simulink model "PruebaSDRRX"  (R2025b)
settings: Solver=VariableStepAuto  StartTime=0.0  StopTime=30  RelTol=1e-3
undefined symbols (not defined in the file or in its folder): gray, RX, TX
libraries: commdigbbndpm3 x1, commfilt2 x1, commsdrhw_v2 x1
settings Model: Creator=JuanDiego  LastModifiedBy=juand

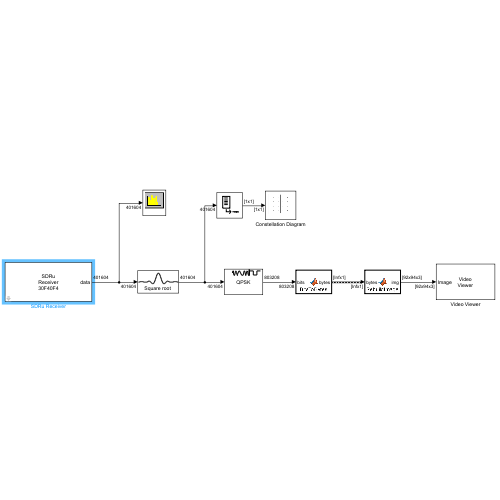
[thumbnail: Simulink's stored preview of the top-level diagram]
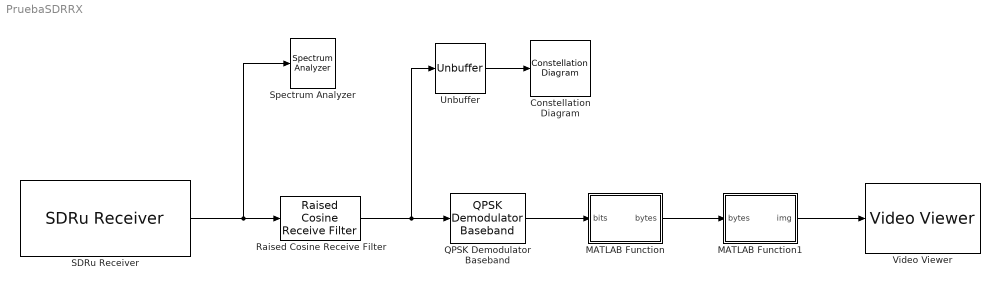
== system PruebaSDRRX ==
  Constellation Diagram : ConstellationDiagram  WindowPosition=[695.000000,130.000000,600.000000,582.000000,]  ScopeFrameLocation=window  SymbolsToDisplaySource=Property  SymbolsToDisplay=5000  ReferenceConstellation=QPSK
  MATLAB Function : MATLAB Function  TreatAsAtomicUnit=on
  MATLAB Function1 : MATLAB Function  TreatAsAtomicUnit=on
  QPSK Demodulator Baseband : commdigbbndpm3/QPSK Demodulator Baseband  OutType=Bit  DecType=Hard decision  VarSource=Dialog  Variance=1  Dec=Gray  Ph=pi/4  outDtype1=double  outDtype2=Inherit via internal rule  derotateFactorWordLen=16  derotateFactorDataTypeStr=Inherit: Same word length as input  derotateFactorLastDataTypeStr=Inherit: Same word length as input
  Raised Cosine Receive Filter : commfilt2/Raised Cosine Receive Filter  filtType=Square root  R=0.25  filtSpan=8  N=8  downFactor=1  downOffset=0  filterGain=1  InputProcessing=Columns as channels (frame based)  RateOptions=Enforce single-rate processing  framing=Mute  checkCoeff=off  variableName=rcRxFilt  currentFiltSpan=10  D=5  inputOffset=0  sampMode=Mute  saveAsFlag=0  rateMode=Downsampling  checkGain=Normalized  launchFVT=on  roundingMode=Floor  overflowMode=off  coeffDataTypeStr=Inherit: Same word length as input  coeffMin=[]  coeffMax=[]  coeffLastDataTypeStr=Inherit: Same word length as input  accumDataTypeStr=Inherit: Same as product output  accumLastDataTypeStr=Inherit: Same as product output  outputDataTypeStr=Inherit: Same as accumulator  outputMin=[]  outputMax=[]  outputLastDataTypeStr=Inherit: Same as accumulator
      settings: LibrarySourceBlock=|
      | commhdlfilt/Raised Cosine
      | Receive Filter
  SDRu Receiver : commsdrhw_v2/SDRu Receiver  rxtx=rx  initializeIPAddress=0  devMap=10  USRP2_IP=192.168.10.2  USRP_IP_X300=192.168.10.2  USRP_IP_X310=192.168.10.2  USRP_IP_N300=192.168.10.2  USRP_IP_N310=192.168.10.2  USRP_IP_N320=192.168.10.2  USRP_IP_E320=192.168.10.2  USRP_IP_X410=192.168.10.2  USRP_serialNumB200=3136D21  USRP_serialNumB210=30F40F4  platform=B210  prevPlatform=B210  lastIPAddressPopup=192.168.10.2  USRP_ID=30F40F4  LastIPAddress=192.168.10.2  IsTwinRXDaughterboard=off  EnableTwinRXPhaseSync=off  losrc=0  ChannelMapping=1  rxAntennaPort=TX/RX  rxAntennaPortX410=RX1  centerFrequencySrc=Dialog  centerFrequency=0.9e9  loOffsetSrc=Dialog  loOffset=0  gainSrc=Dialog  gain=45  PPSSource=Internal  clockSource=Internal  EnableGPSLock=off  EnsureSyncGPSTime=off  EnableTimeTrigger=off  triggerTime=5  enableMIMOCableSync=off  EnableRefLock=off  masterClkRateParam=32000000  masterClkRateB200=32e6  masterClkRateB210=32e6  masterClkRateX300=200e6  masterClkRateX310=200e6  masterClkRateN300=125e6  masterClkRateN310=125e6  masterClkRateN320=200e6  masterClkRateE320=30.72e6  masterClkRateX410=250e6  masterClkRate=100e6  masterClkRateTwinRX=200e6  decimInterpSrc=Dialog  decimInterpPort=512  lastDecimSource=Dialog  decimInterp=32  USRP2_IP_NUM=[51 48 70 52 48 70 52]  sampleRate=1000000  sampleTime=(32)/32000000  TransportDataType=int16  overrunUnderrunPort=off  dataLengthPort=off  EnableTimeStamps=off  outputDatatype=double  frameLength=401604  HOST_DATA_PORT=0  HOST_CONTROL_PORT=0  USRP2_DATA_PORT=0  USRP2_CONTROL_PORT=0  bufferMode=Continuous streaming  EnableBurstMode=off  NumFramesInBurst=207552
  Spectrum Analyzer : SpectrumAnalyzer  WindowPosition=[-1.000000,211.000000,800.000000,500.000000,]  ScopeFrameLocation=window  WindowInvariantSamplesPerUpdate=on  Span=2000000.0000000002  StartFrequency=-1000000.0000000001  StopFrequency=1000000.0000000001  YLimits=[-194.2141 -104.6527]
  Unbuffer : Unbuffer
  Video Viewer : VideoViewer  colormapValue=gray(256)  FigPos=[1 814 1536 717]
  wires:
  SDRu Receiver/1 -> Spectrum Analyzer/1, Raised Cosine Receive Filter/1
  QPSK Demodulator Baseband/1 -> MATLAB Function/1(bits)
  MATLAB Function1/1(img) -> Video Viewer/1
  MATLAB Function/1(bytes) -> MATLAB Function1/1(bytes)
  Raised Cosine Receive Filter/1 -> Unbuffer/1, QPSK Demodulator Baseband/1
  Unbuffer/1 -> Constellation Diagram/1

== matlab function PruebaSDRRX/MATLAB Function ==
  data: bits input; bytes output
function bytes = BitsToBytes(bits)

bits = bits(:);

N = floor(length(bits)/8);

bits = bits(1:8*N);

bits_matrix = reshape(bits,8,[])';

bytes = uint8(bi2de(bits_matrix,'left-msb'));

end

== matlab function PruebaSDRRX/MATLAB Function1 ==
  data: bytes input; img output
function img = RebuildImage(bytes)
filas = 92;
columnas = 94;
canales = 3;
N = filas*columnas*canales;
bytes = uint8(bytes(:));
if length(bytes) < N
    img = zeros(filas,columnas,canales,'uint8');
    return;
end
img = reshape(bytes(1:N),...
              filas,...
              columnas,...
              canales);
end
